simulink model "ex3"  (R2017a)
settings: Solver=VariableStepAuto  StartTime=0.0  StopTime=tf  RelTol=1e-7
undefined symbols (not defined in the file): dt, x0
settings Model: Creator=bruno  LastModifiedBy=bruno

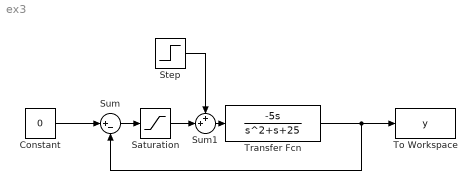
== system ex3 ==
  Constant : Constant  Value=0
  Saturation : Saturate  UpperLimit=1  LowerLimit=-1
  Step : Step  Time=dt  Before=x0/(5*dt)  After=0  SampleTime=0
  Sum : Sum  Inputs=|+-
  Sum1 : Sum  Inputs=++|
  To Workspace : ToWorkspace  VariableName=y  SaveFormat=Structure With Time  SampleTime=-1
  Transfer Fcn : TransferFcn  Numerator=[-5 0]  Denominator=[1 1 25]  ContinuousStateAttributes='Oscilator'
  wires:
  Constant/1 -> Sum/1
  Sum/1 -> Saturation/1
  Transfer Fcn/1 -> Sum/2, To Workspace/1
  Saturation/1 -> Sum1/2
  Sum1/1 -> Transfer Fcn/1
  Step/1 -> Sum1/1
